simulink model "Modele_pour_quatre_quadrants"  (R2015a)
settings: Solver=ode3  StartTime=0.0  StopTime=0.2  FixedStep=1e-5  RelTol=1e-3
values from neighbouring files (symbols this model uses):
  B = 4    [param.m]
  fv = 20    [param.m]
  kprim = (kprim_c+kprim_e)/2    (= 25.4347394903)    [param.m]
  L = 0    [param.m]
  meq = Jeq*i^2/R^2    (= 2.25096401036)    [param.m]
  r = 5.1    [param.m]
  Vsat = 10    [param.m]
libraries: simulink x1
settings Model: Creator=Fred  LastModifiedBy=ASUS
settings SolverCC: ZeroCrossControl=EnableAll  ZeroCrossAlgorithm=Adaptive
settings DebuggingCC: MaxConsecutiveZCsMsg=none

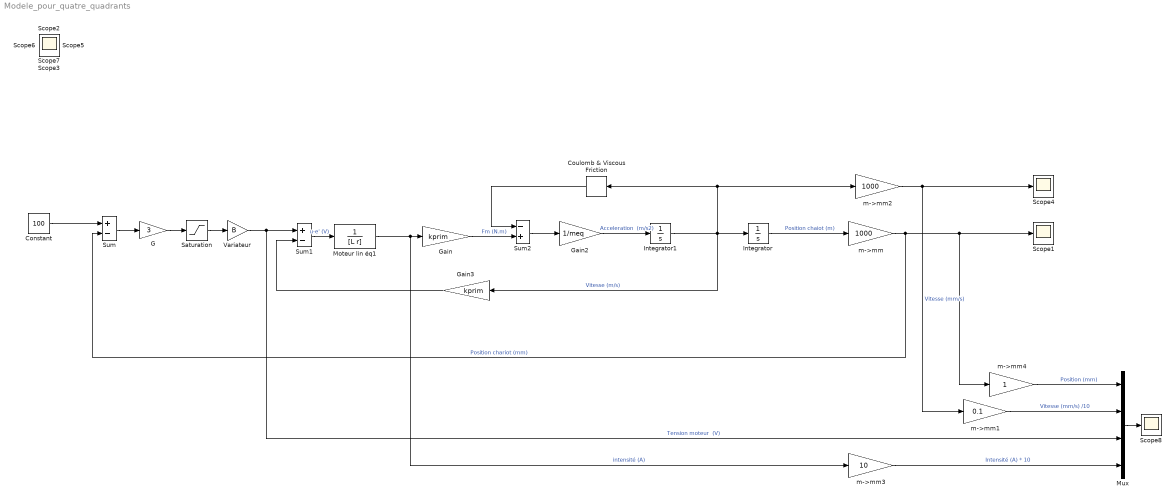
== system Modele_pour_quatre_quadrants ==
  Constant : Constant  Value=100
  Coulomb & Viscous Friction : simulink/Discontinuities/Coulomb & Viscous Friction  offset=Ffrott  gain=fv
  G : Gain  Gain=3
  Gain : Gain  Gain=kprim
  Gain2 : Gain  Gain=1/meq
  Gain3 : Gain  Gain=kprim
  Integrator : Integrator
  Integrator1 : Integrator
  Moteur lin éq1 : TransferFcn  Denominator=[L r]
  Mux : Mux
  Saturation : Saturate  UpperLimit=Vsat  LowerLimit=-Vsat
  Scope{,1..8} (9 alike) : Scope
      Scope1 settings: YMin=-20  YMax=120
      Scope4 settings: TimeRange=5  YMin=1128.232655023233  YMax=1177.551674411152  SaveName=ScopeData4
      Scope8 settings: ShowLegends=on  YMin=-200  YMax=150  SaveName=ScopeData8
      Scope settings: YMin=9  YMax=11
      Scope2 settings: SaveName=ScopeData2
      Scope3 settings: SaveName=ScopeData3
      Scope5 settings: SaveName=ScopeData5
      Scope6 settings: SaveName=ScopeData6
      Scope7 settings: SaveName=ScopeData7
  Sum : Sum  Inputs=+-
  Sum1 : Sum  Inputs=+-
  Sum2 : Sum  Inputs=-+
  Variateur : Gain  Gain=B
  m->mm : Gain  Gain=1000
  m->mm1 : Gain  Gain=0.1
  m->mm2 : Gain  Gain=1000
  m->mm3 : Gain  Gain=10
  m->mm4 : Gain
  wires:
  Sum/1 -> G/1
  Constant/1 -> Sum/1
  G/1 -> Saturation/1
  Gain/1 -> Sum2/2  "Fm (N.m)"
  Gain2/1 -> Integrator1/1  "Acceleration  (m/s2)"
  Sum2/1 -> Gain2/1
  Moteur lin éq1/1 -> m->mm3/1, Gain/1  "intensité (A)"
  Sum1/1 -> Moteur lin éq1/1  "u-e' (V)"
  Integrator1/1 -> m->mm2/1, Coulomb & Viscous Friction/1, Gain3/1, Integrator/1  "Vitesse (m/s)"
  Variateur/1 -> Mux/3, Sum1/1  "Tension moteur  (V)"
  m->mm/1 -> Sum/2, m->mm4/1, Scope1/1  "Position chariot (mm)"
  Coulomb & Viscous Friction/1 -> Sum2/1
  Gain3/1 -> Sum1/2
  Integrator/1 -> m->mm/1  "Position chaiot (m)"
  Saturation/1 -> Variateur/1
  m->mm2/1 -> m->mm1/1, Scope4/1  "Vitesse (mm/s)"
  m->mm1/1 -> Mux/2  "Vitesse (mm/s) /10"
  Mux/1 -> Scope8/1
  m->mm3/1 -> Mux/4  "Intensité (A) * 10"
  m->mm4/1 -> Mux/1  "Position (mm)"
